simulink model "SensingSubsystem_revB"  (R2021b)
settings: Solver=VariableStepAuto  StartTime=0.0  StopTime=stop_time  RelTol=1e-3
values from neighbouring files (symbols this model uses):
  threshold = 15    [sensing_system_revA_performance_evaluation.m]
undefined symbols (not defined in the file or in its folder): chirp_tracking, frame_tracking, max_num_clusters, peak_detection_params, plot_params, spectogram_params, victim
libraries: hdlsllib x4, simulink x3, dspindex x3, dspsigops x2, radarlib x1, dspxfrm3 x1, phasedwavlib x1, dspswit3 x1
settings Model: SimulationMode=accelerator  Creator=David  LastModifiedBy=David

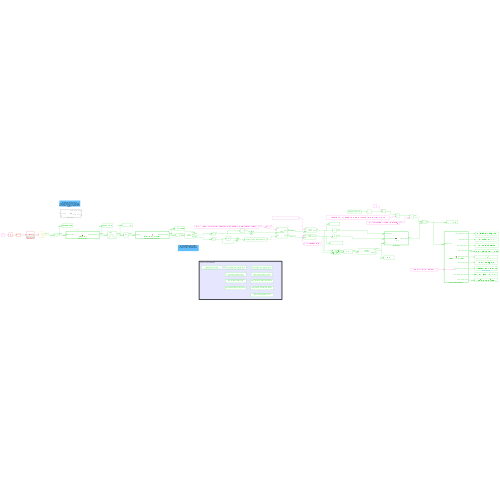
[thumbnail: Simulink's stored preview of the top-level diagram]
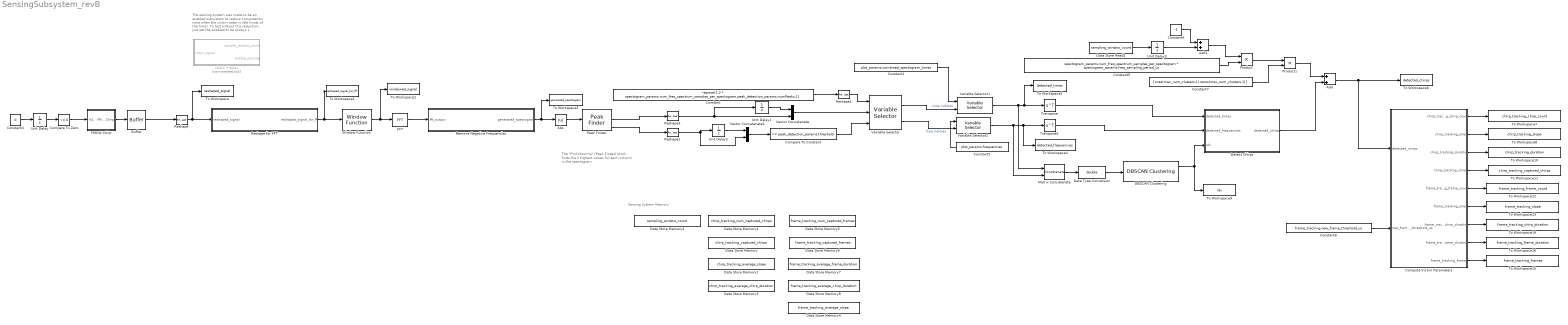
== system SensingSubsystem_revB ==
  note: Sensing System Memory
  note: The sensing system was made to be an enabled subsystem to reduce computation time when the victim radar is idle (most of the time). To test without this reduction, just set the enabled to be always 1
  note: The "Find Maxima" (Peak Finder)
      | block finds the 2 highest values
      | for each column in the spectogram
  Abs : Abs
  Add : Sum
  Add1 : Sum
  Buffer : Buffer  N=int16(spectogram_params.num_ADC_samples_per_spectogram)  OutputFrames=off
  Compare To Constant : simulink/Logic and Bit Operations/Compare To Constant  relop=>=  const=peak_detection_params.threshold  OutDataTypeStr=boolean
  Compare To Zero : simulink/Logic and Bit Operations/Compare To Zero  relop=~=  OutDataTypeStr=boolean
  Compute Victim Parameters : MATLAB Function  TreatAsAtomicUnit=on
  Constant : Constant  Value=repmat(1:2 * spectogram_params.num_freq_spectrum_samples_per_spectogram,peak_detection_params.numPeaks,1)  VectorParams1D=off  OutDataTypeStr=uint32
  Constant1 : Constant  Value=plot_params.combined_spectogram_times
  Constant2 : Constant  Value=plot_params.frequencies
  Constant4 : Constant  Value=0
  Constant5 : Constant  Value=spectogram_params.num_freq_spectrum_samples_per_spectogram * spectogram_params.freq_sampling_period_us
  Constant6 : Constant  Value=-1
  Constant7 : Constant  Value=[ones(max_num_clusters,1),zeros(max_num_clusters,1)]
  Constant8 : Constant  Value=frame_tracking.new_frame_threshold_us
  DBSCAN Clustering : radarlib/DBSCAN Clustering  BlockOutputs=Index and Cluster ID  EpsilonSource=Property  Epsilon=5  MinNumPoints=2  MaxNumPoints=10  EpsilonHistoryLength=10  EnableDisambiguation=off  AmbiguousDimension=1  SimulateUsing=Interpreted execution
      settings: SourceProductBaseCode=RA
  Data Store Memory : DataStoreMemory  DataStoreName=chirp_tracking_captured_chirps  ReadBeforeWriteMsg=warning  WriteAfterWriteMsg=warning  WriteAfterReadMsg=warning  InitialValue=zeros(chirp_tracking.captured_chirps_buffer_size, 2)  ShowAdditionalParam=off  OutDataTypeStr=double
  Data Store Memory1 : DataStoreMemory  DataStoreName=chirp_tracking_average_slope  ReadBeforeWriteMsg=warning  WriteAfterWriteMsg=warning  WriteAfterReadMsg=warning  ShowAdditionalParam=off  OutDataTypeStr=double
  Data Store Memory2 : DataStoreMemory  DataStoreName=sampling_window_count  ReadBeforeWriteMsg=warning  WriteAfterWriteMsg=warning  WriteAfterReadMsg=warning  InitialValue=-1  VectorParams1D=off  ShowAdditionalParam=off  OutDataTypeStr=int16
  Data Store Memory3 : DataStoreMemory  DataStoreName=chirp_tracking_average_chirp_duration  ReadBeforeWriteMsg=warning  WriteAfterWriteMsg=warning  WriteAfterReadMsg=warning  InitialValue=20  ShowAdditionalParam=off  OutDataTypeStr=double
  Data Store Memory4 : DataStoreMemory  DataStoreName=chirp_tracking_num_captured_chirps  ReadBeforeWriteMsg=warning  WriteAfterWriteMsg=warning  WriteAfterReadMsg=warning  ShowAdditionalParam=off  OutDataTypeStr=int16
  Data Store Memory5 : DataStoreMemory  DataStoreName=frame_tracking_num_captured_frames  ReadBeforeWriteMsg=warning  WriteAfterWriteMsg=warning  WriteAfterReadMsg=warning  ShowAdditionalParam=off  OutDataTypeStr=int16
  Data Store Memory6 : DataStoreMemory  DataStoreName=frame_tracking_captured_frames  ReadBeforeWriteMsg=warning  WriteAfterWriteMsg=warning  WriteAfterReadMsg=warning  InitialValue=zeros(frame_tracking.captured_frames_buffer_size,7)  ShowAdditionalParam=off  OutDataTypeStr=double
  Data Store Memory7 : DataStoreMemory  DataStoreName=frame_tracking_average_frame_duration  ReadBeforeWriteMsg=warning  WriteAfterWriteMsg=warning  WriteAfterReadMsg=warning  ShowAdditionalParam=off  OutDataTypeStr=double
  Data Store Memory8 : DataStoreMemory  DataStoreName=frame_tracking_average_chirp_duration  ReadBeforeWriteMsg=warning  WriteAfterWriteMsg=warning  WriteAfterReadMsg=warning  ShowAdditionalParam=off  OutDataTypeStr=double
  Data Store Memory9 : DataStoreMemory  DataStoreName=frame_tracking_average_slope  ReadBeforeWriteMsg=warning  WriteAfterWriteMsg=warning  WriteAfterReadMsg=warning  ShowAdditionalParam=off  OutDataTypeStr=double
  Data Store Read2 : DataStoreRead  DataStoreName=sampling_window_count  IndexOptions=Index vector (dialog)  Indices=1  OutputSizes=1
  Data Type Conversion : DataTypeConversion  OutDataTypeStr=double
  Detect Chirps : MATLAB Function  TreatAsAtomicUnit=on
  FFT : dspxfrm3/FFT  FFTImplementation=Auto  CompMethod=Table lookup  TableOpt=NEW  TableOptActive=Speed  BitRevOrder=off  Normalize=off  InheritFFTLength=on  FFTLength=64  WrapInput=on  roundingMode=Floor  overflowMode=off  firstCoeffDataTypeStr=Inherit: Same word length as input  firstCoeffLastDataTypeStr=Inherit: Same word length as input  outputMin=[]  outputMax=[]
  FMCW Chirp : Subsystem
  Matrix Concatenate : Concatenate  Mode=Multidimensional array  ConcatenateDimension=2
  Peak Finder : dspsigops/Peak Finder  polarity=Maxima  indexBase=One  outputIdx=on  outputVal=on  maxPeaks=peak_detection_params.numPeaks  NoiseDistinguish=off  thresh=1  roundingMode=Floor  overflowMode=off
      settings: SourceProductBaseCode=DS  allowOverrides=off
  Product : Product
  Product1 : Product
  Remove Negative Frequencies : MATLAB Function  TreatAsAtomicUnit=on
  Reshape : Reshape  OutputDimensionality=Customize  OutputDimensions=[spectogram_params.num_ADC_samples_per_spectogram / spectogram_params.num_freq_spectrum_samples_per_spectogram, spectogram_params.num_freq_spectrum_samples_per_spectogram]
  Reshape for FFT : MATLAB Function  TreatAsAtomicUnit=on
  Reshape1 : Reshape
  Reshape2 : Reshape
  Reshape3 : Reshape
  To Workspace : ToWorkspace  VariableName=reshaped_signal  SampleTime=-1
      settings: MaxDataPoints=2
  To Workspace1 : ToWorkspace  VariableName=reshaped_signal_for_fft  SampleTime=-1
      settings: MaxDataPoints=2
  To Workspace10 : ToWorkspace  VariableName=chirp_tracking_duration  SampleTime=-1
      settings: MaxDataPoints=2
  To Workspace11 : ToWorkspace  VariableName=chirp_tracking_captured_chirps  SampleTime=-1
      settings: MaxDataPoints=2
  To Workspace12 : ToWorkspace  VariableName=frame_tracking_frame_count  SampleTime=-1
      settings: MaxDataPoints=2
  To Workspace13 : ToWorkspace  VariableName=frame_tracking_slope  SampleTime=-1
      settings: MaxDataPoints=2
  To Workspace14 : ToWorkspace  VariableName=frame_tracking_chirp_duration  SampleTime=-1
      settings: MaxDataPoints=2
  To Workspace15 : ToWorkspace  VariableName=frame_tracking_frames  SampleTime=-1
      settings: MaxDataPoints=2
  To Workspace16 : ToWorkspace  VariableName=frame_tracking_frame_duration  SampleTime=-1
      settings: MaxDataPoints=2
  To Workspace2 : ToWorkspace  VariableName=windowed_signal  SampleTime=-1
      settings: MaxDataPoints=2
  To Workspace3 : ToWorkspace  VariableName=generated_spectogram  SampleTime=-1
      settings: MaxDataPoints=2
  To Workspace4 : ToWorkspace  VariableName=detected_frequencies  SampleTime=-1
      settings: MaxDataPoints=2
  To Workspace5 : ToWorkspace  VariableName=detected_times  SampleTime=-1
      settings: MaxDataPoints=2
  To Workspace6 : ToWorkspace  VariableName=detected_chirps  SampleTime=-1
      settings: MaxDataPoints=2
  To Workspace7 : ToWorkspace  VariableName=chirp_tracking_chirp_count  SampleTime=-1
      settings: MaxDataPoints=2
  To Workspace8 : ToWorkspace  VariableName=chirp_tracking_slope  SampleTime=-1
      settings: MaxDataPoints=2
  To Workspace9 : ToWorkspace  VariableName=idx  SampleTime=-1
      settings: MaxDataPoints=2
  Transpose : Math  Operator=transpose  SaturateOnIntegerOverflow=on
  Transpose1 : Math  Operator=transpose  SaturateOnIntegerOverflow=on
  Unit Delay : UnitDelay  InitialCondition=1  SampleTime=-1  HasFrameUpgradeWarning=on
  Unit Delay1 : UnitDelay  SampleTime=-1  HasFrameUpgradeWarning=on
  Unit Delay2 : UnitDelay  SampleTime=-1  HasFrameUpgradeWarning=on
  Unit Delay3 : UnitDelay  SampleTime=-1  HasFrameUpgradeWarning=on
  Variable Selector : dspindex/Variable Selector  NumInputs=2  rowsOrCols=Columns  IdxMode=Variable  Elements=[1 3]  ZerOneIdxMode=One-based  errmode=Clip Index  FillMode=on  FillValues=0
  Variable Selector1 : dspindex/Variable Selector  NumInputs=1  rowsOrCols=Rows  IdxMode=Variable  Elements=[1 3]  ZerOneIdxMode=One-based  errmode=Clip Index  FillMode=off  FillValues=0
  Variable Selector2 : dspindex/Variable Selector  NumInputs=1  rowsOrCols=Rows  IdxMode=Variable  Elements=[1 3]  ZerOneIdxMode=One-based  errmode=Clip Index  FillMode=off  FillValues=0
  Vector Concatenate : Concatenate
  Vector Concatenate1 : Concatenate
  Window Function : dspsigops/Window Function  winmode=Apply window to input  wintype=Hann  sampmode=Continuous  samptime=1  N=64  Rs=50  beta=10  winsamp=Symmetric  UserWindow=hamming  OptParams=off  UserParams={'symmetric'}  dataType=double  isSigned=on  wordLen=16  udDataType=sfix(16)  fracBitsMode=Best precision  numFracBits=15  roundingMode=Floor  overflowMode=off  numSidelobes=4  sidelobeLevel=-30
      settings: SourceProductBaseCode=DS
  check if zeros : MATLAB Function  Commented=on  TreatAsAtomicUnit=on
  wires:
  Unit Delay/1 -> Compare To Zero/1
  Compare To Zero/1 -> FMCW Chirp/1(In1)
  Constant4/1 -> Unit Delay/1
  FMCW Chirp/1(FMCW Chirp) -> Buffer/1
  Variable Selector/2 -> Variable Selector2/2  "freq indicies"
  Compute Victim Parameters/7(frame_tracking_chirp_duration) -> To Workspace14/1
  Reshape2/1 -> Vector Concatenate1/2, Unit Delay2/1
  Abs/1 -> Peak Finder/1
  Constant7/1 -> Product1/2
  Window Function/1 -> FFT/1, To Workspace2/1
  Remove Negative Frequencies/1(generated_spectogram) -> Abs/1, To Workspace3/1
  Add/1 -> Compute Victim Parameters/1(detected_chirps), To Workspace6/1
  Variable Selector2/1 -> Matrix Concatenate/2, To Workspace4/1, Transpose1/1
  Matrix Concatenate/1 -> Data Type Conversion/1
  Reshape3/1 -> Vector Concatenate/2, Unit Delay1/1
  Transpose1/1 -> Detect Chirps/2(detected_frequencies)
  Product/1 -> Product1/1
  Compute Victim Parameters/5(frame_tracking_frame_count) -> To Workspace12/1
  Data Store Read2/1 -> Unit Delay3/1
  Compute Victim Parameters/2(chirp_tracking_slope) -> To Workspace8/1
  Peak Finder/3 -> Reshape2/1
  Peak Finder/2 -> Reshape3/1
  Constant6/1 -> Add1/1
  Reshape1/1 -> Variable Selector/1
  Constant5/1 -> Product/2
  Transpose/1 -> Detect Chirps/1(detected_times)
  FFT/1 -> Remove Negative Frequencies/1(fft_output)
  Product1/1 -> Add/1
  Compute Victim Parameters/1(chirp_tracking_chirp_count) -> To Workspace7/1
  Vector Concatenate/1 -> Variable Selector/2
  Detect Chirps/1(detected_chirps) -> Add/2
  Reshape for FFT/1(reshaped_signal_for_fft) -> Window Function/1, To Workspace1/1
  Constant1/1 -> Variable Selector1/1
  Constant2/1 -> Variable Selector2/1
  Variable Selector/1 -> Variable Selector1/2  "time indicies"
  Vector Concatenate1/1 -> Compare To Constant/1
  Compute Victim Parameters/4(chirp_tracking_chirps) -> To Workspace11/1
  Unit Delay1/1 -> Vector Concatenate/1
  Unit Delay2/1 -> Vector Concatenate1/1
  Compare To Constant/1 -> Variable Selector/3
  Data Type Conversion/1 -> DBSCAN Clustering/1
  Compute Victim Parameters/9(frame_tracking_frames) -> To Workspace15/1
  Variable Selector1/1 -> Matrix Concatenate/1, To Workspace5/1, Transpose/1
  Buffer/1 -> Reshape/1
  Reshape/1 -> Reshape for FFT/1(reshaped_signal), To Workspace/1
  Constant8/1 -> Compute Victim Parameters/2(new_frame_threshold_us)
  Compute Victim Parameters/3(chirp_tracking_duration) -> To Workspace10/1
  Compute Victim Parameters/6(frame_tracking_slope) -> To Workspace13/1
  Constant/1 -> Reshape1/1
  DBSCAN Clustering/1 -> To Workspace9/1, Detect Chirps/3(idx)
  Compute Victim Parameters/8(frame_tracking_frame_duration) -> To Workspace16/1
  Add1/1 -> Product/1
  Unit Delay3/1 -> Add1/2

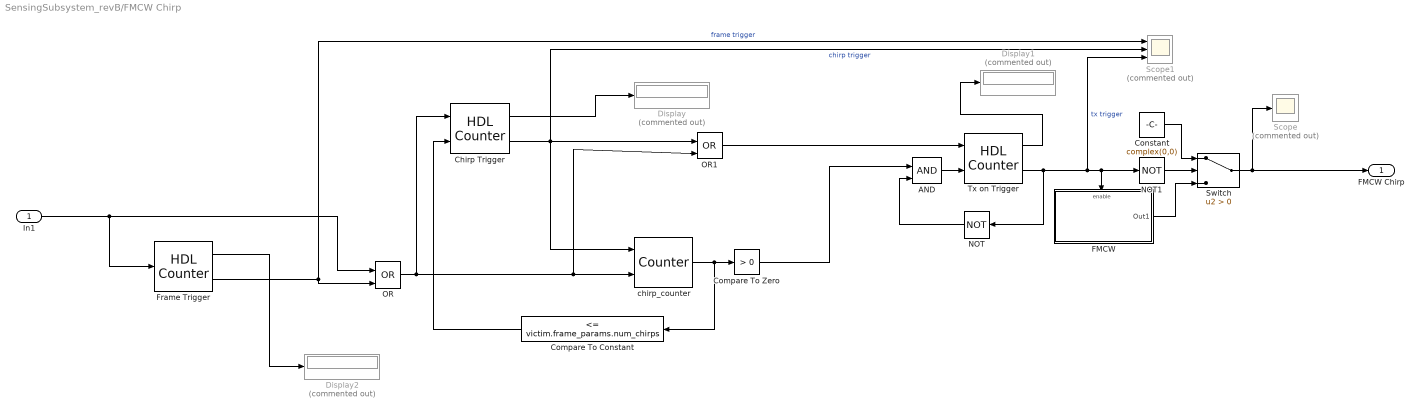
== system SensingSubsystem_revB/FMCW Chirp ==
  In1 : Inport
  AND : Logic  IconShape=distinctive  AllPortsSameDT=off  OutDataTypeStr=boolean
  Chirp Trigger : hdlsllib/Sources/HDL Counter  CountType=Count limited  CountInit=1  CountStep=1  CountMax=victim.waveform_params.sample_rate_Hz * victim.waveform_params.sweep_time_s + victim.chirp_params.num_samples_idle_time  CountFromType=Initial value  CountFrom=1  CountResetPort=on  CountLoadPort=off  CountEnbPort=on  CountDirPort=off  CountHitOutputPort=on  CountDataType=Unsigned  CountWordLen=16  CountFracLen=0  CountSampTime=1
  Compare To Constant : simulink/Logic and Bit Operations/Compare To Constant  relop=<=  const=victim.frame_params.num_chirps  OutDataTypeStr=boolean
  Compare To Zero : hdlsllib/Logic and Bit Operations/Compare To Zero  relop=>  OutDataTypeStr=boolean
      settings: SourceProductBaseCode=SL
  Constant : Constant  Value=complex(0,0)
  Display : Display  Commented=on
  Display1 : Display  Commented=on
  Display2 : Display  Commented=on
  FMCW : Subsystem
  Frame Trigger : hdlsllib/Sources/HDL Counter  CountType=Count limited  CountInit=1  CountStep=1  CountMax=victim.frame_params.num_samples_per_frame  CountFromType=Initial value  CountFrom=1  CountResetPort=on  CountLoadPort=off  CountEnbPort=off  CountDirPort=off  CountHitOutputPort=on  CountDataType=Unsigned  CountWordLen=32  CountFracLen=0  CountSampTime=1
  NOT : Logic  Operator=NOT  IconShape=distinctive  AllPortsSameDT=off  OutDataTypeStr=boolean
  NOT1 : Logic  Operator=NOT  IconShape=distinctive  AllPortsSameDT=off  OutDataTypeStr=boolean
  OR : Logic  Operator=OR  IconShape=distinctive  AllPortsSameDT=off  OutDataTypeStr=boolean
  OR1 : Logic  Operator=OR  IconShape=distinctive  AllPortsSameDT=off  OutDataTypeStr=boolean
  Scope : Scope  Commented=on
  Scope1 : Scope  Commented=on  NumInputPorts=3
  Switch : Switch  Criteria=u2 > Threshold
  Tx on Trigger : hdlsllib/Sources/HDL Counter  CountType=Count limited  CountInit=1  CountStep=1  CountMax=victim.chirp_params.num_samples_idle_time  CountFromType=Initial value  CountFrom=1  CountResetPort=on  CountLoadPort=off  CountEnbPort=on  CountDirPort=off  CountHitOutputPort=on  CountDataType=Unsigned  CountWordLen=16  CountFracLen=0  CountSampTime=1
  chirp_counter : dspswit3/Counter  Direction=Up  CountEvent=Rising edge  CounterSize=User defined  MaxCount=victim.frame_params.num_chirps + 1  InitialCount=1  Output=Count  HitValue=32  ResetInput=on  SamplesPerFrame=1  Ts=1  CntDtype=int16  HitDtype=Logical
  FMCW Chirp : Outport
  wires:
  Switch/1 -> FMCW Chirp/1, Scope/1
  chirp_counter/1 -> Compare To Constant/1, Compare To Zero/1
  Tx on Trigger/2 -> NOT/1, Scope1/3, FMCW/Enable, NOT1/1  "tx trigger"
  AND/1 -> Tx on Trigger/2
  FMCW/1(Out1) -> Switch/3
  NOT1/1 -> Switch/2
  Constant/1 -> Switch/1
  Chirp Trigger/1 -> Display/1
  Chirp Trigger/2 -> chirp_counter/1, OR1/1, Scope1/2  "chirp trigger"
  Compare To Zero/1 -> AND/1
  NOT/1 -> AND/2
  Compare To Constant/1 -> Chirp Trigger/2
  Frame Trigger/2 -> OR/2, Scope1/1  "frame trigger"
  Tx on Trigger/1 -> Display1/1
  Frame Trigger/1 -> Display2/1
  In1/1 -> Frame Trigger/1, OR/1
  OR/1 -> Chirp Trigger/1, OR1/2, chirp_counter/2
  OR1/1 -> Tx on Trigger/1

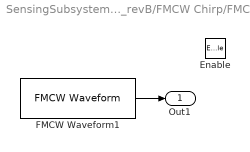
== system SensingSubsystem_revB/FMCW Chirp/FMCW ==
  Enable : EnablePort  StatesWhenEnabling=reset
  FMCW Waveform1 : phasedwavlib/FMCW Waveform  SampleRate=victim.waveform_params.sample_rate_Hz  SweepTime=victim.waveform_params.sweep_time_s  SweepBandwidth=victim.waveform_params.sweep_BW_Hz  SweepDirection=Up  SweepInterval=Positive  OutputFormat=Samples  NumSamples=1  NumSweeps=waveform_params.num_sweeps  SimulateUsing=Interpreted execution
      settings: SourceProductBaseCode=AR
  Out1 : Outport
  wires:
  FMCW Waveform1/1 -> Out1/1

== matlab function SensingSubsystem_revB/Remove Negative Frequencies ==
  data: fft_output input; generated_spectogram output; half_fft_size parameter
function generated_spectogram = remove_negative_frequencies(fft_output, half_fft_size)
   
generated_spectogram = fft_output(1:half_fft_size,:);

== matlab function SensingSubsystem_revB/Reshape for FFT ==
  data: reshaped_signal input; reshaped_signal_for_fft output; fft_size parameter
function reshaped_signal_for_fft = reshape_for_fft(reshaped_signal, fft_size)
   
reshaped_signal_for_fft = reshaped_signal(1:fft_size,:);

== matlab function SensingSubsystem_revB/Detect Chirps ==
  data: detected_times input; detected_chirps output; detected_frequencies input; idx input; max_num_clusters parameter; sampling_window_count data_store_memory; threshold parameter
function detected_chirps  = detect_chirps(detected_times,detected_frequencies,idx,max_num_clusters,threshold)
    %solve for the linear equation for each cluster provided there are enough
    %points
    detected_chirps = zeros(max_num_clusters,2);
    global sampling_window_count;
    for cluster_id = 1:max(idx)
        %solve for linear model using linear algrebra
        %y is frequencies, x is time
        if sum(idx == cluster_id) > threshold && all(detected_times(idx == cluster_id))
            X = [ones(size(detected_times(idx == cluster_id),2),1),detected_times(idx == cluster_id).'];
            Y = detected_frequencies(idx == cluster_id).';
            B = inv(X.' * X) * X.' * Y;
            detected_chirps(cluster_id,1:2) = [-B(1)/B(2),B(2)];
        end
    end
%    sampling_window_count = sampling_window_count + 1;
end

== matlab function SensingSubsystem_revB/Compute Victim Parameters ==
  data: detected_chirps input; chirp_tracking_average_chirp_duration data_store_memory; chirp_tracking_captured_chirps data_store_memory; chirp_tracking_average_slope data_store_memory; chirp_tracking_num_captured_chirps data_store_memory; chirp_tracking_chirp_count output; chirp_tracking_slope output; chirp_tracking_duration output; chirp_tracking_chirps output; new_frame_threshold_us input; frame_tracking_num_captured_frames data_store_memory; frame_tracking_captured_frames data_store_memory; frame_tracking_average_frame_duration data_store_memory; frame_tracking_average_chirp_duration data_store_memory; frame_tracking_average_slope data_store_memory; sampling_window_count data_store_memory; frame_tracking_frame_count output; frame_tracking_slope output; frame_tracking_chirp_duration output; frame_tracking_frame_duration output; frame_tracking_frames output; captured_chirps_buffer_size parameter
function [chirp_tracking_chirp_count, chirp_tracking_slope, chirp_tracking_duration, chirp_tracking_chirps,...
    frame_tracking_frame_count,frame_tracking_slope,frame_tracking_chirp_duration,frame_tracking_frame_duration, frame_tracking_frames] ...
    = compute_victim_parameters(detected_chirps, new_frame_threshold_us, captured_chirps_buffer_size)
    

    %declare global variables for accessing previously captured chirps, the
    %previously computed chirp duration, and the average slope

    %chirp tracking global variables
    global chirp_tracking_average_chirp_duration chirp_tracking_average_slope chirp_tracking_captured_chirps chirp_tracking_num_captured_chirps;

    %frame tracking global variables
    global frame_tracking_num_captured_frames frame_tracking_captured_frames frame_tracking_average_frame_duration frame_tracking_average_chirp_duration frame_tracking_average_slope
    
    %for tracking the sampling window
    global sampling_window_count

    for i = 1:size(detected_chirps,1)
        if detected_chirps(i,2) ~= 0 && chirp_tracking_num_captured_chirps < captured_chirps_buffer_size
            if chirp_tracking_num_captured_chirps == 0 %if the captured chirps buffer is empty (i.e: first chirp detected or first chirp in a frame)
                chirp_tracking_captured_chirps(1,:) = detected_chirps(i,:);
                chirp_tracking_num_captured_chirps = chirp_tracking_num_captured_chirps + 1;                
            elseif all(abs(chirp_tracking_captured_chirps - detected_chirps(i,1)) > chirp_tracking_average_chirp_duration / 2,'all')
                if chirp_tracking_num_captured_chirps >= 2
                    duration_difference_from_avg = abs(detected_chirps(i,1) - chirp_tracking_captured_chirps(chirp_tracking_num_captured_chirps,1) - chirp_tracking_average_chirp_duration);
                    if duration_difference_from_avg >= new_frame_threshold_us %declare as part of a new frame
                        %increment the frame counter
                        frame_tracking_num_captured_frames = frame_tracking_num_captured_frames + 1;
                        %save the duration, number of chirps, average slope, average chirp duration, start time, and sampling window count
                        frame_tracking_captured_frames(frame_tracking_num_captured_frames,1) = detected_chirps(i,1) - chirp_tracking_captured_chirps(1,1);  % duration
                        frame_tracking_captured_frames(frame_tracking_num_captured_frames,2) = chirp_tracking_num_captured_chirps;                          % number of chirps
                        frame_tracking_captured_frames(frame_tracking_num_captured_frames,3) = chirp_tracking_average_slope;                                % average slope
                        frame_tracking_captured_frames(frame_tracking_num_captured_frames,4) = chirp_tracking_average_chirp_duration;                       % average_chirp_duration
                        frame_tracking_captured_frames(frame_tracking_num_captured_frames,5) = chirp_tracking_captured_chirps(1,1);
                        frame_tracking_captured_frames(frame_tracking_num_captured_frames,6) = sampling_window_count;

                        %reset the chirp tracking
                        chirp_tracking_num_captured_chirps = int16(0);
                        chirp_tracking_captured_chirps = zeros(captured_chirps_buffer_size, 2);
                        chirp_tracking_average_chirp_duration = 0;
                        chirp_tracking_average_slope = 0; %#ok<NASGU> 
                        
                        %reset sampling window - not implemented yet
                        frame_tracking_average_frame_duration = sum(frame_tracking_captured_frames(:,1)) / double(frame_tracking_num_captured_frames);
                        
                        %compute the overall averages for chirp slope
                        %and duration
                        frame_tracking_average_chirp_duration =  ...
                            sum(frame_tracking_captured_frames(:,4) .* (frame_tracking_captured_frames(:,2) - 1))/ ...
                            sum((frame_tracking_captured_frames(frame_tracking_captured_frames(:,2) ~=0,2) - 1));
                        frame_tracking_average_slope = ...
                            sum(frame_tracking_captured_frames(:,3) .* (frame_tracking_captured_frames(:,2) - 1))/ ...
                            sum((frame_tracking_captured_frames(frame_tracking_captured_frames(:,2) ~=0,2) - 1));

                        %compute the predicted time for the next chirp
                        %to occur on.
                        frame_tracking_captured_frames(frame_tracking_num_captured_frames,7) = ...
                                    detected_chirps(i,1) + frame_tracking_average_frame_duration;
                    end
                end
                chirp_tracking_captured_chirps(chirp_tracking_num_captured_chirps + 1,:) = detected_chirps(i,:);
                chirp_tracking_num_captured_chirps = chirp_tracking_num_captured_chirps + 1;

            end
            chirp_tracking_average_slope = sum(chirp_tracking_captured_chirps(1:chirp_tracking_num_captured_chirps,2))/ ...
                double(chirp_tracking_num_captured_chirps);
            if chirp_tracking_num_captured_chirps >= 2
                chirp_tracking_average_chirp_duration = (chirp_tracking_captured_chirps(chirp_tracking_num_captured_chirps,1) - ...
                    chirp_tracking_captured_chirps(1,1))/double(chirp_tracking_num_captured_chirps - 1);
            end
        end
    end

    %output the new parameters for reference
    chirp_tracking_chirp_count = chirp_tracking_num_captured_chirps;
    chirp_tracking_slope = chirp_tracking_average_slope;
    chirp_tracking_duration = chirp_tracking_average_chirp_duration;
    chirp_tracking_chirps = chirp_tracking_captured_chirps;

    frame_tracking_frame_count = frame_tracking_num_captured_frames;
    frame_tracking_slope = frame_tracking_average_slope;
    frame_tracking_chirp_duration = frame_tracking_average_chirp_duration;
    frame_tracking_frame_duration = frame_tracking_average_frame_duration;
    frame_tracking_frames = frame_tracking_captured_frames;

    sampling_window_count = sampling_window_count + 1;
end

== matlab function SensingSubsystem_revB/check if zeros ==
  data: sample_window_count output; input_signal input; enable_sensing output; sampling_window_count data_store_memory
function [sample_window_count,enable_sensing] = fcn(input_signal)
    global sampling_window_count
    if ~all(input_signal == 0,"all")
        enable_sensing = 1;
    else
        enable_sensing = 0;
        if sampling_window_count > 0
            sampling_window_count = sampling_window_count + 1;
        end
    end
    sample_window_count = sampling_window_count;
end
